simulink model "set_throttle"  (R2020a)
settings: Solver=FixedStepDiscrete  StartTime=0.0  StopTime=10.0  RelTol=1e-3
settings Model: Creator=thomas  LastModifiedBy=thomas

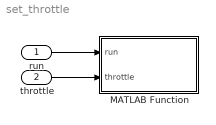
== system set_throttle ==
  run : Inport  OutDataTypeStr=boolean
  throttle : Inport  Port=2  OutDataTypeStr=double
  MATLAB Function : MATLAB Function  TreatAsAtomicUnit=on
  wires:
  throttle/1 -> MATLAB Function/2(throttle)
  run/1 -> MATLAB Function/1(run)

== matlab function set_throttle/MATLAB Function ==
  data: run input; throttle input
function set_throttle(run, throttle)
    coder.extrinsic('evalin');
    if run
        evalin('base', sprintf('vessel_control.setThrottle(%0.5f);', throttle));
    end
end
